simulink model "daniel_modelos"  (R2016a)
settings: Solver=VariableStepAuto  StartTime=0.0  StopTime=50  MaxStep=0.01  RelTol=1e-3
values from neighbouring files (symbols this model uses):
  A = [0 1  0              0 ... (first row only)    [MatLab4p.m]    (also in MatLab5p.m = [     0        1       0        0; MatLab6p.m = [     0        1       0        0; _Labs.m = [     0        1       0        0; q2.m = [0 1  0   0)
  Am = blkdiag(M,M)    [MatLab5p.m]    (also in MatLab6p.m; _Labs.m; q2.m = 1; questao2.m = 1)
  B = [0; 1/M; 0; -1/(M*L)]    [MatLab4p.m]    (also in MatLab5p.m = [ 0    0; MatLab6p.m = [ 0    0; _Labs.m = [ 0    0; q2.m = [  0)
  Bm = blkdiag(N,N)    [MatLab5p.m]    (also in MatLab6p.m; _Labs.m; q2.m = N; questao2.m = N)
  C = [1 0 0 0]    [MatLab4p.m]    (also in MatLab5p.m = [1 0 0 0; MatLab6p.m = [1 0 0 0; _Labs.m = [1 0 0 0; q2.m)
  Cm = eye(1)    [q2.m]    (also in questao2.m = eye(3))
  Dm = zeros(1,1)    [q2.m]    (also in questao2.m = zeros(3,1))
  Dsim = zeros(4,1)    [MatLab4p.m]    (also in MatLab5p.m = zeros(4,2); MatLab6p.m = zeros(4,2); _Labs.m = zeros(4,2); q2.m)
  K = place(A,B,[-2 -2.05 -2.1 -2.15])    [MatLab4p.m]    (also in MatLab5p.m = Ka(:,1:4); MatLab6p.m = Ka(:,1:4); _Labs.m = Ka(:,1:4); q2.m = Ka(:,1:4))
  Kl = kd*inv(T)    [questao2.m]
  Km = Ka(:,5:10)    [MatLab5p.m]    (also in MatLab6p.m; _Labs.m; q2.m = Ka(5); questao2.m = Ka(:,5:7))
  L = (place(A',C',[-6 -6.05 -6.1 -6.15]))'    [MatLab4p.m]    (also in MatLab6p.m = H'; _Labs.m = H'; q2.m = H'; questao2.m = H')
  x0 = [0 0 pi/4 0]    [MatLab4p.m]    (also in MatLab5p.m = [1 0.5 1 0.1]; MatLab6p.m = [1 2 0.8 -0.3]; _Labs.m = [1 2 0.8 -0.3]; q2.m = [0 0 pi/6 0])
  x0obs = [0.05 0 pi/5 0]    [MatLab4p.m]    (also in MatLab6p.m = [0 0 0 0]; _Labs.m = [0 0 0 0]; questao2.m = [0 0 0 0])
settings Model: Creator=Regner  LastModifiedBy=Regner

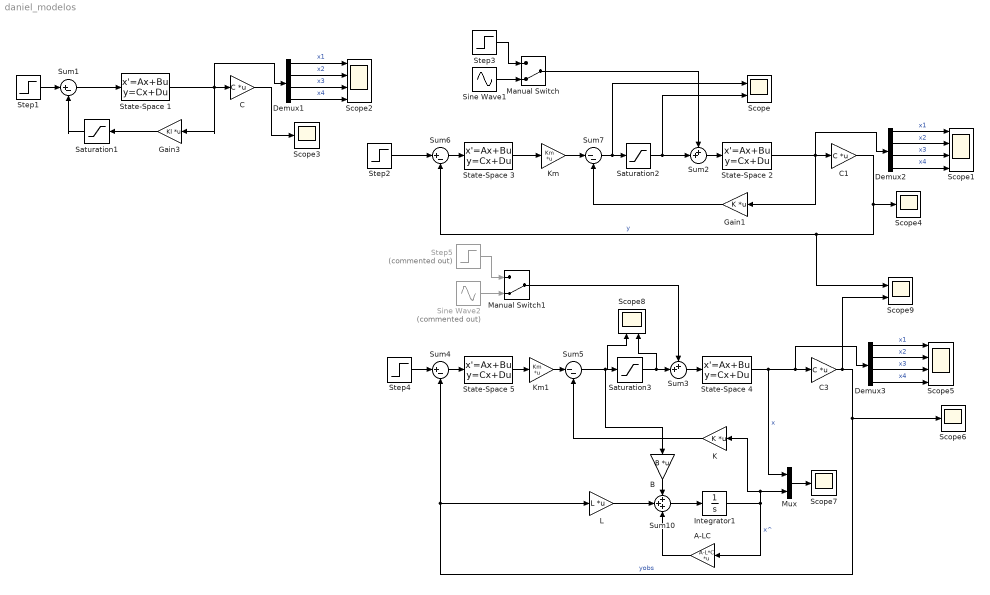
== system daniel_modelos ==
  A-LC : Gain  Gain=A-L*C  Multiplication=Matrix(K*u)
  B : Gain  Gain=B  Multiplication=Matrix(K*u)
  C : Gain  Gain=C  Multiplication=Matrix(K*u)
  C1 : Gain  Gain=C  Multiplication=Matrix(K*u)
  C3 : Gain  Gain=C  Multiplication=Matrix(K*u)
  Demux1 : Demux
  Demux2 : Demux
  Demux3 : Demux
  Gain1 : Gain  Gain=K  Multiplication=Matrix(K*u)
  Gain3 : Gain  Gain=Kl  Multiplication=Matrix(K*u)
  Integrator1 : Integrator  InitialCondition=x0obs
  K : Gain  Gain=K  Multiplication=Matrix(K*u)
  Km : Gain  Gain=Km  Multiplication=Matrix(K*u)
  Km1 : Gain  Gain=Km  Multiplication=Matrix(K*u)
  L : Gain  Gain=L  Multiplication=Matrix(K*u)
  Manual Switch : ManualSwitch  CurrentSetting=0
  Manual Switch1 : ManualSwitch  CurrentSetting=0
  Mux : Mux  Inputs=2
  Saturation1 : Saturate  UpperLimit=50  LowerLimit=-50
  Saturation2 : Saturate  UpperLimit=50  LowerLimit=-50  ZeroCross=off
  Saturation3 : Saturate  UpperLimit=50  LowerLimit=-50  ZeroCross=off
  Scope : Scope  NumInputPorts=2
  Scope1 : Scope  NumInputPorts=4
  Scope2 : Scope  NumInputPorts=4
  Scope{3..4,6..7} (4 alike) : Scope
  Scope5 : Scope  NumInputPorts=4
  Scope8 : Scope  NumInputPorts=2
  Scope9 : Scope  NumInputPorts=2
  Sine Wave1 : Sin  Amplitude=10  Frequency=0.1  SampleTime=0
  Sine Wave2 : Sin  Commented=on  Amplitude=10  Frequency=0.1  SampleTime=0
  State-Space 1 : StateSpace  A=A  B=B  C=eye(4)  D=Dsim  X0=x0
  State-Space 2 : StateSpace  A=A  B=B  C=eye(4)  D=Dsim  X0=x0
  State-Space 3 : StateSpace  A=Am  B=Bm  C=Cm  D=Dm  X0=0
  State-Space 4 : StateSpace  A=A  B=B  C=eye(4)  D=Dsim  X0=x0
  State-Space 5 : StateSpace  A=Am  B=Bm  C=Cm  D=Dm  X0=0
  Step1 : Step  Time=0  After=0  SampleTime=0
  Step2 : Step  Time=0  After=0  SampleTime=0
  Step3 : Step  Time=10  After=pi  SampleTime=0
  Step4 : Step  Time=0  After=0  SampleTime=0
  Step5 : Step  Commented=on  Time=10  After=0  SampleTime=0
  Sum1 : Sum  Inputs=|+-
  Sum10 : Sum  Inputs=+++
  Sum2 : Sum  Inputs=++|
  Sum3 : Sum  Inputs=++|
  Sum4 : Sum  Inputs=|+-
  Sum5 : Sum  Inputs=|--
  Sum6 : Sum  Inputs=|+-
  Sum7 : Sum  Inputs=|--
  wires:
  Demux1/1 -> Scope2/1  "x1"
  Demux1/2 -> Scope2/2  "x2"
  Demux1/3 -> Scope2/3  "x3"
  Demux1/4 -> Scope2/4  "x4"
  C/1 -> Scope3/1
  State-Space 1/1 -> C/1, Demux1/1, Gain3/1
  Step1/1 -> Sum1/1
  Sum1/1 -> State-Space 1/1
  Gain3/1 -> Saturation1/1
  Saturation1/1 -> Sum1/2
  Demux3/1 -> Scope5/1  "x1"
  Demux3/2 -> Scope5/2  "x2"
  Demux3/3 -> Scope5/3  "x3"
  Demux3/4 -> Scope5/4  "x4"
  State-Space 4/1 -> C3/1, Demux3/1, Mux/1  "x"
  Step4/1 -> Sum4/1
  Sum4/1 -> State-Space 5/1
  K/1 -> Sum5/2
  State-Space 5/1 -> Km1/1
  Km1/1 -> Sum5/1
  Sum3/1 -> State-Space 4/1
  Sum5/1 -> Scope8/1, B/1, Saturation3/1
  Demux2/1 -> Scope1/1  "x1"
  Demux2/2 -> Scope1/2  "x2"
  Demux2/3 -> Scope1/3  "x3"
  Demux2/4 -> Scope1/4  "x4"
  C1/1 -> Scope9/1, Sum6/2, Scope4/1  "y"
  State-Space 2/1 -> Gain1/1, Demux2/1, C1/1
  Step2/1 -> Sum6/1
  Sum6/1 -> State-Space 3/1
  Gain1/1 -> Sum7/2
  State-Space 3/1 -> Km/1
  Km/1 -> Sum7/1
  Sum2/1 -> State-Space 2/1
  Manual Switch/1 -> Sum2/1
  Sum7/1 -> Scope/1, Saturation2/1
  Saturation2/1 -> Sum2/2, Scope/2
  Saturation3/1 -> Sum3/2, Scope8/2
  C3/1 -> Scope9/2, Sum4/2, L/1, Scope6/1  "yobs"
  Sum10/1 -> Integrator1/1
  L/1 -> Sum10/2
  A-LC/1 -> Sum10/3
  Integrator1/1 -> K/1, Mux/2, A-LC/1  "x^"
  B/1 -> Sum10/1
  Mux/1 -> Scope7/1
  Sine Wave1/1 -> Manual Switch/2
  Step3/1 -> Manual Switch/1
  Manual Switch1/1 -> Sum3/1
  Sine Wave2/1 -> Manual Switch1/2
  Step5/1 -> Manual Switch1/1
